simulink model "rotpentemplateV3"  (R2021b)
settings: Solver=ode45  StartTime=0.0  StopTime=run_time  RelTol=1e-3  EnableMultiTasking=on
values from neighbouring files (symbols this model uses):
  adingain = [adingain 1 1 1 1 1]    [hwinit.m]
  adinoffs = [adinoffs 0 0 0 0 0]    [hwinit.m]
  daoutgain = 1*[-6]    [hwinit.m]
  daoutoffs = [0.00]    [hwinit.m]
  h = 0.01    [Multisine_test.m]    (also in animate_pendulum.m = mean(diff(t)); collect_arm2_freeswing.m; collect_freeswing.m; first-script.m)
  K = lqr(A, B, Q, R)    [compute_lqr.m]    (also in link2_ode.m = zeros(2, 1); run_controller.m = K_full; run_ref_tracking.m = K_full(1:4))
  ref = [-pi; 0; 0; 0]    [run_controller.m]    (also in run_lqr.m = [pi; 0; 0; 0]; run_mpc.m = [pi; 0]; run_ref_tracking.m = ref_eq)
settings Model: Creator=rbabuska  LastModifiedBy=tvanzelderen
settings SolverCC: AlgebraicLoopSolver=TrustRegion
settings DataIOCC: LimitDataPoints=on  SaveFormat=Array  ReturnWorkspaceOutputs=off  SignalLoggingName=sigsOut
settings OptimizationCC: BooleanDataType=off  ExpressionDepthLimit=2147483647  InitFltsAndDblsToZero=on  LifeSpan=inf
settings DebuggingCC: SaveWithParameterizedLinksMsg=none  SignalResolutionControl=TryResolveAllWithWarning  MultiTaskDSMMsg=warning  MultiTaskCondExecSysMsg=none  AllowSymbolicDim=off  StateNameClashWarn=warning  SFUnexpectedBacktrackingDiag=warning  SFNoUnconditionalDefaultTransitionDiag=warning  SFExecutionAtInitializationDiag=none  ArithmeticOperatorsInVariantConditions=warning
settings HardwareCC: ProdBitPerPointer=32  ProdBitPerSizeT=32  ProdBitPerPtrDiffT=32  ProdLargestAtomicFloat=None  ProdIntDivRoundTo=Undefined  ProdEndianess=Unspecified  ProdWordSize=32  ProdHWDeviceType=32-bit Generic  TargetUnknown=on
settings ModelReferenceCC: PropagateSignalLabelsOutOfModel=off
settings SFSimCC: SimUseLocalCustomCode=off  CustomCodeUndefinedFunction=UseInterfaceOnly
settings RTWCC: RTWUseLocalCustomCode=off
settings CodeAppCC: StateflowObjectComments=on
settings GRTTargetCC: TargetFcnLib=ansi_tfl_tmw.mat  TargetLangStandard=C89/C90 (ANSI)  CombineOutputUpdateFcns=off  GRTInterface=on
settings ConfigComp: CovMetricSettings=dw  CovSaveCumulativeToWorkspaceVar=on  CovSaveSingleToWorkspaceVar=on  CovExternalEMLEnable=off

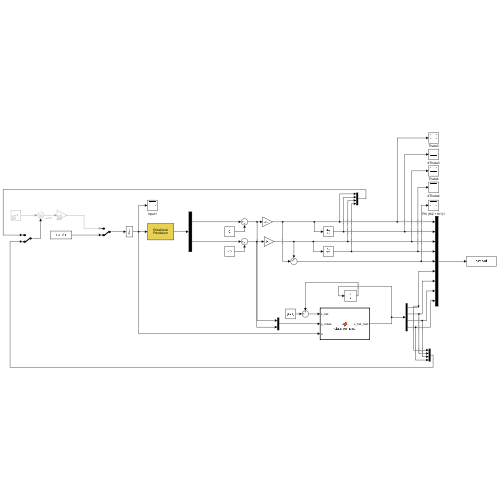
[thumbnail: Simulink's stored preview of the top-level diagram]
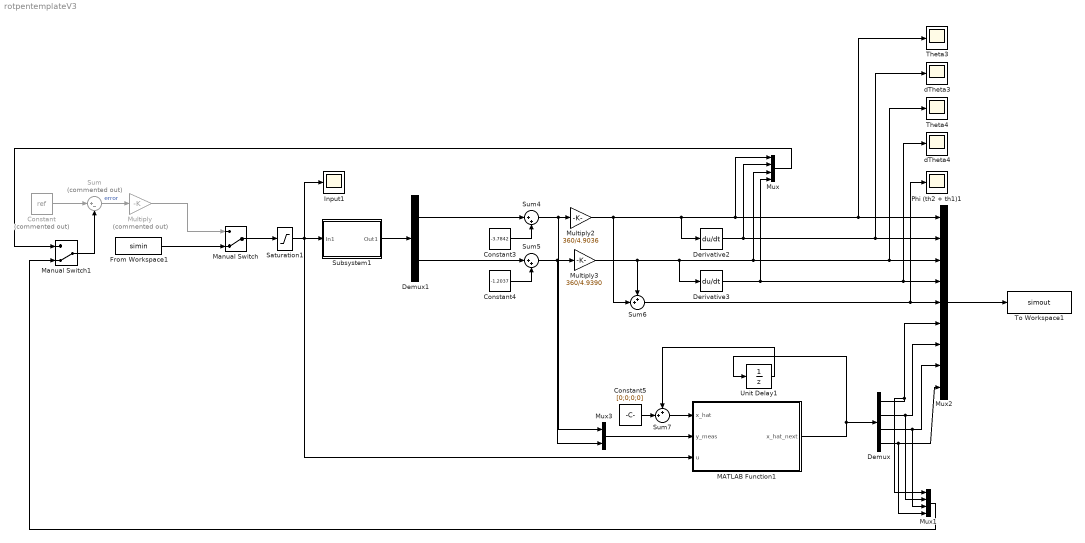
== system rotpentemplateV3 ==
  Constant : Constant  Commented=on  Value=ref
  Constant3 : Constant  Value=-3.7842
  Constant4 : Constant  Value=-1.2037
  Constant5 : Constant  Value=[0;0;0;0]
  Demux : Demux
  Demux1 : Demux  Outputs=2
  Derivative2 : Derivative
  Derivative3 : Derivative
  From Workspace1 : FromWorkspace  VariableName=simin
  Input1 : Scope
  MATLAB Function1 : MATLAB Function  TreatAsAtomicUnit=on
  Manual Switch : ManualSwitch  CurrentSetting=0
  Manual Switch1 : ManualSwitch  CurrentSetting=0
  Multiply : Gain  Commented=on  Gain=-K
  Multiply2 : Gain  Gain=360/4.9036
  Multiply3 : Gain  Gain=360/4.9390
  Mux : Mux
  Mux1 : Mux
  Mux2 : Mux  Inputs=9
  Mux3 : Mux  Inputs=2
  Phi (th2 + th1)1 : Scope
  Saturation1 : Saturate  UpperLimit=1  LowerLimit=-1
  Subsystem1 : Subsystem
      mask Display: disp('Rotational\nPendulum')
  Sum : Sum  Commented=on  Inputs=|+-
  Sum4 : Sum  Inputs=|++
  Sum5 : Sum  Inputs=|++
  Sum6 : Sum  Inputs=++|
  Sum7 : Sum  Inputs=++|
  Theta3 : Scope
  Theta4 : Scope
  To Workspace1 : ToWorkspace  VariableName=simout  SaveFormat=Timeseries  SampleTime=-1
  Unit Delay1 : UnitDelay  SampleTime=0.01  HasFrameUpgradeWarning=on
  dTheta3 : Scope
  dTheta4 : Scope
  wires:
  Mux3/1 -> MATLAB Function1/2(y_meas)
  Derivative3/1 -> Mux/4, dTheta4/1, Mux2/4
  Unit Delay1/1 -> Sum7/1
  Sum6/1 -> Phi (th2 + th1)1/1, Mux2/5
  Constant3/1 -> Sum4/2
  Mux2/1 -> To Workspace1/1
  Sum5/1 -> Multiply3/1, Mux3/2
  Sum4/1 -> Mux3/1, Multiply2/1
  Demux1/1 -> Sum4/1
  MATLAB Function1/1(x_hat_next) -> Demux/1, Unit Delay1/1
  Constant4/1 -> Sum5/2
  Demux1/2 -> Sum5/1
  Sum7/1 -> MATLAB Function1/1(x_hat)
  Saturation1/1 -> Subsystem1/1(In1), Input1/1, MATLAB Function1/3(u)
  Multiply3/1 -> Theta4/1, Mux2/3, Mux/3, Derivative3/1, Sum6/1
  Multiply2/1 -> Theta3/1, Mux2/1, Mux/1, Derivative2/1, Sum6/2
  Derivative2/1 -> dTheta3/1, Mux2/2, Mux/2
  Constant5/1 -> Sum7/2
  Subsystem1/1(Out1) -> Demux1/1
  Demux/1 -> Mux1/1, Mux2/6
  Demux/2 -> Mux1/2, Mux2/7
  Demux/3 -> Mux1/3, Mux2/8
  Demux/4 -> Mux1/4, Mux2/9
  Constant/1 -> Sum/1
  Sum/1 -> Multiply/1  "error"
  Multiply/1 -> Manual Switch/1
  From Workspace1/1 -> Manual Switch/2
  Manual Switch/1 -> Saturation1/1
  Mux1/1 -> Manual Switch1/2
  Mux/1 -> Manual Switch1/1
  Manual Switch1/1 -> Sum/2

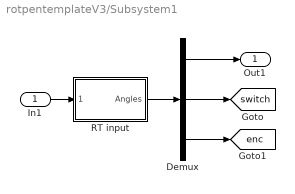
== system rotpentemplateV3/Subsystem1 ==
  In1 : Inport
  Demux : Demux  Outputs=[2 4 1]
  RT input : Subsystem  mask{Ts=h, channels=[6 7]}
      mask prompts: Ts "Sample time [s]:"; channels "Channels to read (e.g., [6 7])"
      mask init:
      | hwinit;
      | 
      | % initialize FPGA
      | fugihandle = fugiboard('Open', 'Pendulum1');
      | fugihandle.WatchdogTimeout = 0.5;
      | fugiboard('SetParams', fugihandle);
      | fugiboard('Write', fugihandle, 0, 0, 0, 0);  % dummy write to sync interface board
      | fugiboard('Write', fugihandle, 5, 1, 0, 0);  % reset position, activate relay
      | data = fugiboard('Read', fugihandle);        % get version info from FPGA
      | % model = bitshift(data(1), -5); 
      | % version = bitand(data(1), 31);
      | % disp(sprintf('FPGA setup %d, version %d', model, version)); % for the B&P it should say 1 1, or else there is a problem
      | fugiboard('Write', fugihandle, 0, 1, 0, 0);  % end reset
      | pause(0.1);                         % give relay some time to respond
      mask Display: disp('Rotational\nPendulum')
  Out1 : Outport
  tag scope: enc=global, switch=global
  wires:
  RT input/1(Angles) -> Demux/1
  Demux/1 -> Out1/1
  Demux/2 -> [switch]
  Demux/3 -> [enc]
  In1/1 -> RT input/1(Motors)

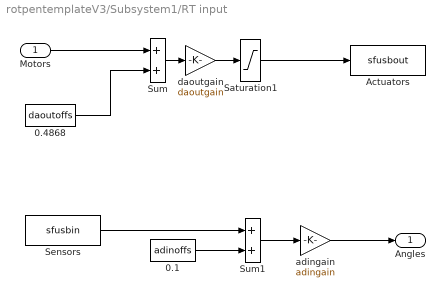
== system rotpentemplateV3/Subsystem1/RT input ==
  Motors : Inport
  0.1 : Constant  Value=adinoffs
  0.4868 : Constant  Value=daoutoffs
  Actuators : S-Function  FunctionName=sfusbout  Parameters=Ts, fugihandle  SFunctionDeploymentMode=off  EnableBusSupport=off
  Saturation1 : Saturate  UpperLimit=10  LowerLimit=-10
  Sensors : S-Function  FunctionName=sfusbin  Parameters=Ts, fugihandle, channels  SFunctionDeploymentMode=off  EnableBusSupport=off
  Sum : Sum  InputSameDT=on  SaturateOnIntegerOverflow=on  OutDataTypeStr=Inherit: Same as first input
  Sum1 : Sum  InputSameDT=on  SaturateOnIntegerOverflow=on  OutDataTypeStr=Inherit: Same as first input
  adingain : Gain  Gain=adingain  SaturateOnIntegerOverflow=on  OutDataTypeStr=Inherit: Same as input  ParamDataTypeStr=Inherit: Same as input
  daoutgain : Gain  Gain=daoutgain  SaturateOnIntegerOverflow=on  OutDataTypeStr=Inherit: Same as input  ParamDataTypeStr=Inherit: Same as input
  Angles : Outport
  wires:
  Sum/1 -> daoutgain/1
  0.4868/1 -> Sum/2
  Motors/1 -> Sum/1
  Sum1/1 -> adingain/1
  0.1/1 -> Sum1/2
  adingain/1 -> Angles/1
  Saturation1/1 -> Actuators/1
  daoutgain/1 -> Saturation1/1
  Sensors/1 -> Sum1/1

== matlab function rotpentemplateV3/MATLAB Function1 ==
  data: x_hat input; y_meas input; u input; x_hat_next output
function x_hat_next = observer_step(x_hat, y_meas, u)
    % 1. Pre-allocate output
    x_hat_next = zeros(4, 1);
    
    % 2. Force inputs to strict column vectors and scalars
    x = reshape(x_hat, 4, 1);
    y = reshape(y_meas, 2, 1);
    u_in = u(1);
    h = 0.001;
    
    % Gain Matrices (Added commas for strict compiler parsing)
    L = [  13.2692,    2.4922;
         -104.1660,  -83.3741;
          -15.9139,    0.9017;
           17.9635,  165.8050];
          
    C = [1, 0, 0, 0;
         0, 0, 1, 0];
         
    % 3. RK4 integration using the sub-function below
    % Innovation (correction) terms
    innov1 = y - C * x;
    k1 = calculate_ode(x, u_in) + L * innov1;
    
    innov2 = y - C * (x + (h/2)*k1);
    k2 = calculate_ode(x + (h/2)*k1, u_in) + L * innov2;
    
    innov3 = y - C * (x + (h/2)*k2);
    k3 = calculate_ode(x + (h/2)*k2, u_in) + L * innov3;
    
    innov4 = y - C * (x + h*k3);
    k4 = calculate_ode(x + h*k3, u_in) + L * innov4;
    
    x_hat_next = x + (h/6)*(k1 + 2*k2 + 2*k3 + k4);
end

% ---------------------------------------------------------
% LOCAL FUNCTION: Flattened for Simulink Compilation
% ---------------------------------------------------------
function dxdt = calculate_ode(x, u)
    % HARDCODE PARAMETERS directly as scalar variables
    l1 = 0.10;                         
    m1 = 0.25;                         
    lc1 = l1 / 2;                     
    J1 = (1/3) * m1 * l1^2;       
    l2 = 0.086841;                     
    m2 = 0.024;                        
    J2 = m2 * l2^2;               
    alpha2 = 0.164111;                   
    c2 = alpha2 * m2 * l2^2;  
    
    % Stable testing parameters (Update after Step Test!)
    km = 18;                      
    kbc1 = 2.5;      %CHANGE THIS               
    g = 9.81;                         
    
    % Unpack states
    th1  = x(1);
    dth1 = x(2);
    th2  = x(3);
    dth2 = x(4);
    
    % Torque
    tau = -km * u;
    
    % Inertia Matrix (M) components broken down for parsing safety
    M11 = J1 + m2*(l1^2 + l2^2 + 2*l1*l2*cos(th2));
    M12 = m2*(l2^2 + l1*l2*cos(th2));
    M21 = m2*(l2^2 + l1*l2*cos(th2));
    M22 = m2*l2^2;
    M = [M11, M12; 
         M21, M22];
    
    % Right-hand side (rhs) components broken down for parsing safety
    h_val = m2*l1*l2*sin(th2);
    
    rhs1 = tau - kbc1*dth1 - (-h_val*(2*dth1*dth2 + dth2^2)) - ((m1*lc1 + m2*l1)*g*sin(th1) + m2*g*l2*sin(th1+th2));
    rhs2 = -c2*dth2 - (h_val*dth1^2) - (m2*g*l2*sin(th1+th2));
    rhs = [rhs1; rhs2];
    
    % Solve for accelerations
    ddq = M \ rhs;
    
    % Pack derivative output
    dxdt = zeros(4, 1);
    dxdt(1) = dth1;
    dxdt(2) = ddq(1);
    dxdt(3) = dth2;
    dxdt(4) = ddq(2);
end
